simulink model "SsmithPredictor"  (R2022b)
settings: Solver=VariableStepAuto  StartTime=0.0  StopTime=Tsim  RelTol=1e-3
values from neighbouring files (symbols this model uses):
  Ampdist = 0.5    [smithPredictor.m]
  L = 2    [smithPredictor.m]
  s = tf('s')    [smithPredictor.m]
  Tdist = 20    [smithPredictor.m]
  Tinit = 5    [smithPredictor.m]
libraries: cstblocks x5, simulink x1
settings Model: Creator=jprmj  LastModifiedBy=jprmj

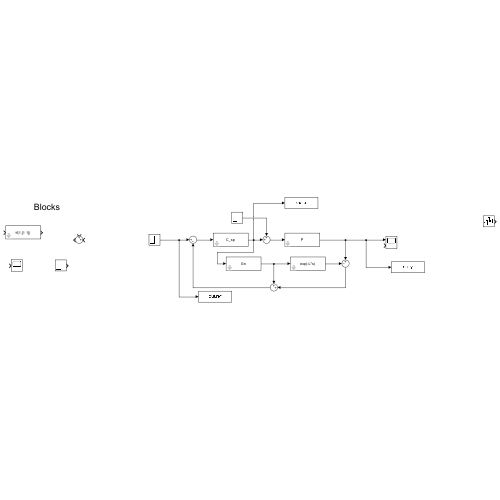
[thumbnail: Simulink's stored preview of the top-level diagram]
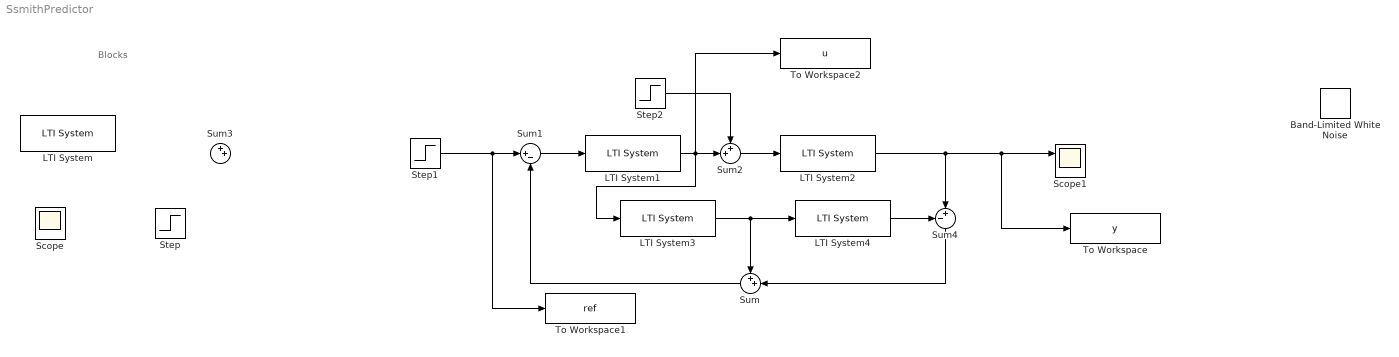
== system SsmithPredictor ==
  note: Blocks
  Band-Limited White Noise : simulink/Sources/Band-Limited White Noise  Cov=[0.1]  Ts=0.1  seed=[23341]
  LTI System : cstblocks/LTI System  sys=tf(1,[1 1])  IC=[]
  LTI System1 : cstblocks/LTI System  sys=C_sp  IC=[]
  LTI System2 : cstblocks/LTI System  sys=P  IC=[]
  LTI System3 : cstblocks/LTI System  sys=Gn  IC=[]
  LTI System4 : cstblocks/LTI System  sys=exp(-L*s)  IC=[]
  Scope : Scope
  Scope1 : Scope  NumInputPorts=2
  Step : Step  SampleTime=0
  Step1 : Step  SampleTime=Tinit
  Step2 : Step  After=Ampdist  SampleTime=Tdist
  Sum : Sum  Inputs=++|
  Sum1 : Sum  Inputs=|+-
  Sum2 : Sum  Inputs=++|
  Sum3 : Sum  Inputs=++|
  Sum4 : Sum  Inputs=-+|
  To Workspace : ToWorkspace  VariableName=y  SaveFormat=Timeseries  SampleTime=-1
  To Workspace1 : ToWorkspace  VariableName=ref  SaveFormat=Timeseries  SampleTime=-1
  To Workspace2 : ToWorkspace  VariableName=u  SaveFormat=Timeseries  SampleTime=-1
  wires:
  LTI System2/1 -> Sum4/2, To Workspace/1, Scope1/1
  Step1/1 -> To Workspace1/1, Sum1/1
  Sum1/1 -> LTI System1/1
  Sum2/1 -> LTI System2/1
  Step2/1 -> Sum2/1
  LTI System1/1 -> LTI System3/1, To Workspace2/1, Sum2/2
  LTI System3/1 -> Sum/1, LTI System4/1
  LTI System4/1 -> Sum4/1
  Sum4/1 -> Sum/2
  Sum/1 -> Sum1/2
